simulink model "linear_2_tank_model"  (R2019b)
settings: Solver=VariableStepAuto  StartTime=0.0  StopTime=10.0  RelTol=1e-3
values from neighbouring files (symbols this model uses):
  xe1 = 4.35641    [script_task_2_linear.m]    (also in script_task_2_nonlinear.m)
  xe2 = 4.47    [script_task_2_linear.m]    (also in script_task_2_nonlinear.m)
settings Model: Creator=NicSch02  LastModifiedBy=NicSch02

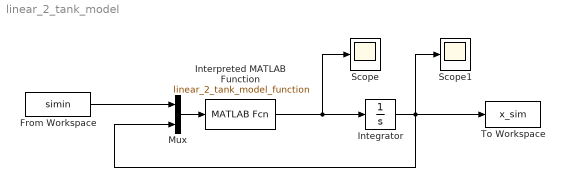
== system linear_2_tank_model ==
  From Workspace : FromWorkspace  VariableName=simin  SampleTime=0
  Integrator : Integrator  InitialCondition=[xe1; xe2;]
  Interpreted MATLAB Function : MATLABFcn  MATLABFcn=linear_2_tank_model_function
  Mux : Mux  Inputs=2
  Scope : Scope
  Scope1 : Scope
  To Workspace : ToWorkspace  VariableName=x_sim  SaveFormat=Structure With Time  SampleTime=-1
  wires:
  Interpreted MATLAB Function/1 -> Scope/1, Integrator/1
  From Workspace/1 -> Mux/1
  Integrator/1 -> Scope1/1, Mux/2, To Workspace/1
  Mux/1 -> Interpreted MATLAB Function/1
